simulink model "LIB_p2d_model_reference_R2021b"  (R2021b)
settings: Solver=FixedStepDiscrete  StartTime=0.0  StopTime=inf  FixedStep=dt  RelTol=1e-3
values from neighbouring files (symbols this model uses):
  Const = 0.065777522687874415    [LIB_p2d_dictionary.sldd]
  MatC = <binary blob, 30483 chars, not shown>    [LIB_p2d_dictionary.sldd]
  n1 = 5.0    [LIB_p2d_dictionary.sldd]    (also in P2D_run.m = mesh.n1)
  n2 = 2.0    [LIB_p2d_dictionary.sldd]    (also in P2D_run.m = mesh.n2)
  n3 = 5.0    [LIB_p2d_dictionary.sldd]    (also in P2D_run.m = mesh.n3)
  n4 = 5.0    [LIB_p2d_dictionary.sldd]
  ord = 2.0    [LIB_p2d_dictionary.sldd]    (also in P2D_run.m = mesh.ord)
undefined symbols (not defined in the file or in its folder): full
settings Model: DataDictionary=LIB_p2d_dictionary.sldd  EnableAccessToBaseWorkspace=off  Creator=simba  LastModifiedBy=simba
settings DebuggingCC: ParameterPrecisionLossMsg=none  UnconnectedInputMsg=none  UnconnectedOutputMsg=none  UnconnectedLineMsg=none
settings ModelReferenceCC: EnableRefExpFcnMdlSchedulingChecks=off
settings RTWCC: GPUComputeCapability=5.0  DLArmComputeVersion=20.02.1
settings ConfigComp: CovBoundaryAbsTol=1.0e-5

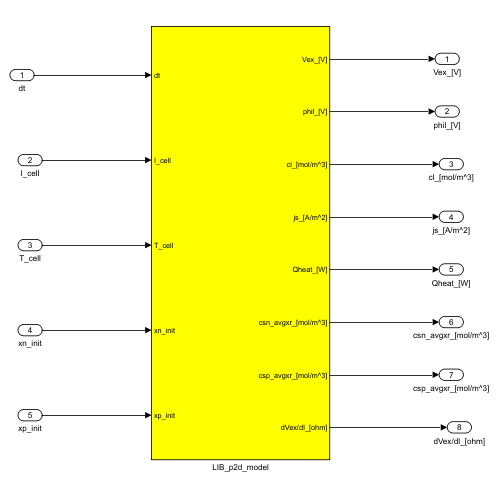
[thumbnail: Simulink's stored preview of the top-level diagram]
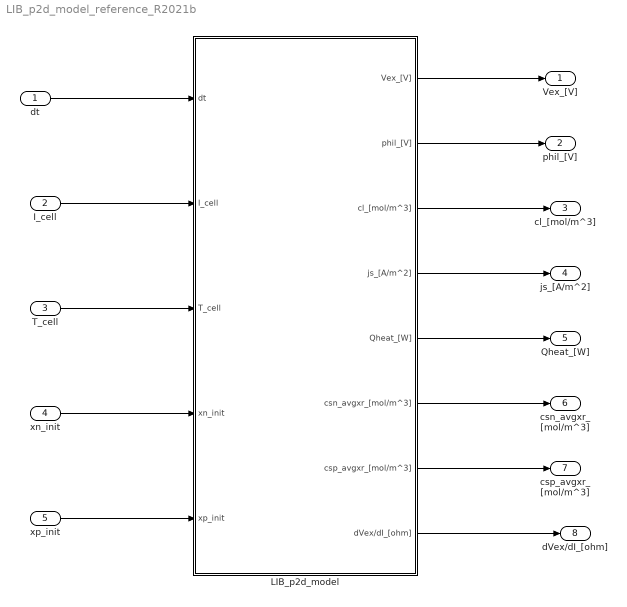
== system LIB_p2d_model_reference_R2021b ==
  dt : Inport  OutDataTypeStr=single
  I_cell : Inport  Port=2  OutDataTypeStr=single
  T_cell : Inport  Port=3  OutDataTypeStr=single
  xn_init : Inport  Port=4  OutDataTypeStr=single
  xp_init : Inport  Port=5  OutDataTypeStr=single
  LIB_p2d_model : Subsystem
  Vex_[V] : Outport
  phil_[V] : Outport  Port=2
  cl_[mol/m^3] : Outport  Port=3
  js_[A/m^2] : Outport  Port=4
  Qheat_[W] : Outport  Port=5
  csn_avgxr_[mol/m^3] : Outport  Port=6
  csp_avgxr_[mol/m^3] : Outport  Port=7
  dVex/dI_[ohm] : Outport  Port=8
  wires:
  dt/1 -> LIB_p2d_model/1(dt)
  I_cell/1 -> LIB_p2d_model/2(I_cell)
  T_cell/1 -> LIB_p2d_model/3(T_cell)
  xn_init/1 -> LIB_p2d_model/4(xn_init)
  xp_init/1 -> LIB_p2d_model/5(xp_init)
  LIB_p2d_model/1(Vex_[V]) -> Vex_[V]/1
  LIB_p2d_model/2(phil_[V]) -> phil_[V]/1
  LIB_p2d_model/3(cl_[mol/m^3]) -> cl_[mol/m^3]/1
  LIB_p2d_model/4(js_[A/m^2]) -> js_[A/m^2]/1
  LIB_p2d_model/5(Qheat_[W]) -> Qheat_[W]/1
  LIB_p2d_model/6(csn_avgxr_[mol/m^3]) -> csn_avgxr_[mol/m^3]/1
  LIB_p2d_model/7(csp_avgxr_[mol/m^3]) -> csp_avgxr_[mol/m^3]/1
  LIB_p2d_model/8(dVex/dI_[ohm]) -> dVex/dI_[ohm]/1

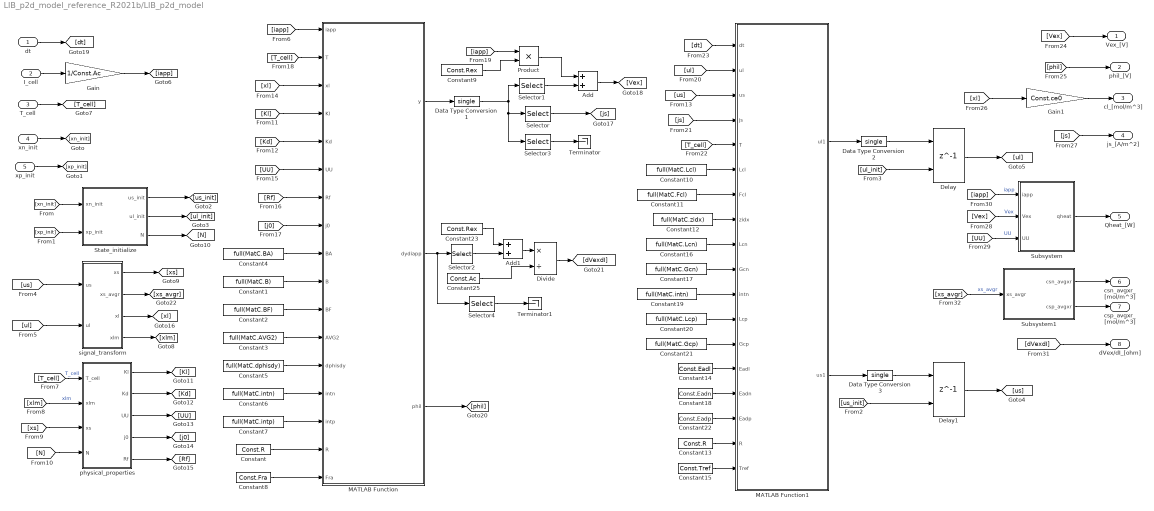
== system LIB_p2d_model_reference_R2021b/LIB_p2d_model ==
  dt : Inport
  I_cell : Inport  Port=2
  T_cell : Inport  Port=3
  xn_init : Inport  Port=4
  xp_init : Inport  Port=5
  Add : Sum
  Add1 : Sum
  Constant : Constant  Value=Const.R  OutDataTypeStr=single
  Constant1 : Constant  Value=full(MatC.B)  OutDataTypeStr=single
  Constant10 : Constant  Value=full(MatC.Lcl)  OutDataTypeStr=single
  Constant11 : Constant  Value=full(MatC.Fcl)  OutDataTypeStr=single
  Constant12 : Constant  Value=full(MatC.zidx)  OutDataTypeStr=uint8
  Constant13 : Constant  Value=Const.R  OutDataTypeStr=single
  Constant14 : Constant  Value=Const.Eadl  OutDataTypeStr=single
  Constant15 : Constant  Value=Const.Tref  OutDataTypeStr=single
  Constant16 : Constant  Value=full(MatC.Lcn)  OutDataTypeStr=single
  Constant17 : Constant  Value=full(MatC.Gcn)  OutDataTypeStr=single
  Constant18 : Constant  Value=Const.Eadn  OutDataTypeStr=single
  Constant19 : Constant  Value=full(MatC.intn)  VectorParams1D=off  OutDataTypeStr=single
  Constant2 : Constant  Value=full(MatC.BF)  OutDataTypeStr=single
  Constant20 : Constant  Value=full(MatC.Lcp)  OutDataTypeStr=single
  Constant21 : Constant  Value=full(MatC.Gcp)  OutDataTypeStr=single
  Constant22 : Constant  Value=Const.Eadp  OutDataTypeStr=single
  Constant23 : Constant  Value=Const.Rex  OutDataTypeStr=single
  Constant25 : Constant  Value=Const.Ac  OutDataTypeStr=single
  Constant3 : Constant  Value=full(MatC.AVG2)  OutDataTypeStr=single
  Constant4 : Constant  Value=full(MatC.BA)  OutDataTypeStr=single
  Constant5 : Constant  Value=full(MatC.dphisdy)  OutDataTypeStr=single
  Constant6 : Constant  Value=full(MatC.intn)  VectorParams1D=off  OutDataTypeStr=single
  Constant7 : Constant  Value=full(MatC.intp)  VectorParams1D=off  OutDataTypeStr=single
  Constant8 : Constant  Value=Const.Fra  OutDataTypeStr=single
  Constant9 : Constant  Value=Const.Rex  OutDataTypeStr=single
  Data Type Conversion1 : DataTypeConversion  OutDataTypeStr=single
  Data Type Conversion2 : DataTypeConversion  OutDataTypeStr=single
  Data Type Conversion3 : DataTypeConversion  OutDataTypeStr=single
  Delay : Delay  DelayLength=1  InitialConditionSource=Input port  InitialCondition=0
      settings: InputPortMap=u0,p4
  Delay1 : Delay  DelayLength=1  InitialConditionSource=Input port  InitialCondition=0
      settings: InputPortMap=u0,p4
  Divide : Product  Inputs=*/
  Gain : Gain  Gain=1/Const.Ac
  Gain1 : Gain  Gain=Const.ce0
  MATLAB Function : MATLAB Function  TreatAsAtomicUnit=on
  MATLAB Function1 : MATLAB Function  TreatAsAtomicUnit=on
  Product : Product
  Selector : Selector  IndexOptions=Index vector (dialog)  Indices=1:n1+n3  OutputSizes=1
  Selector1 : Selector  IndexOptions=Index vector (dialog)  Indices=n1+n3+2  OutputSizes=1
  Selector2 : Selector  IndexOptions=Index vector (dialog)  Indices=n1+n3+2  OutputSizes=1
  Selector3 : Selector  IndexOptions=Index vector (dialog)  Indices=n1+n3+3  OutputSizes=1
  Selector4 : Selector  IndexOptions=Index vector (dialog)  Indices=n1+n3+3  OutputSizes=1
  State_initialize : Subsystem
  Subsystem : Subsystem
  Subsystem1 : Subsystem
  Terminator : Terminator
  Terminator1 : Terminator
  physical_properties : Subsystem
  signal_transform : Subsystem
  Vex_[V] : Outport
  phil_[V] : Outport  Port=2
  cl_[mol/m^3] : Outport  Port=3
  js_[A/m^2] : Outport  Port=4
  Qheat_[W] : Outport  Port=5
  csn_avgxr_[mol/m^3] : Outport  Port=6
  csp_avgxr_[mol/m^3] : Outport  Port=7
  dVex/dI_[ohm] : Outport  Port=8
  wires:
  xn_init/1 -> [xn_init]
  xp_init/1 -> [xp_init]
  [xn_init] -> State_initialize/1(xn_init)
  [xp_init] -> State_initialize/2(xp_init)
  State_initialize/1(us_init) -> [us_init]
  State_initialize/2(ul_init) -> [ul_init]
  [us_init] -> Delay1/2
  [ul_init] -> Delay/2
  [us] -> signal_transform/1(us)
  [ul] -> signal_transform/2(ul)
  I_cell/1 -> Gain/1
  Gain/1 -> [iapp]
  T_cell/1 -> [T_cell]
  signal_transform/4(xlm) -> [xlm]
  [T_cell] -> physical_properties/1(T_cell)  "T_cell"
  [xlm] -> physical_properties/2(xlm)  "xlm"
  signal_transform/1(xs) -> [xs]
  [xs] -> physical_properties/3(xs)
  State_initialize/3(N) -> [N]
  [N] -> physical_properties/4(N)
  physical_properties/1(Kl) -> [Kl]
  physical_properties/2(Kd) -> [Kd]
  physical_properties/3(UU) -> [UU]
  physical_properties/4(j0) -> [j0]
  physical_properties/5(Rf) -> [Rf]
  [iapp] -> MATLAB Function/1(iapp)
  [Kl] -> MATLAB Function/4(Kl)
  Constant4/1 -> MATLAB Function/9(BA)
  Constant1/1 -> MATLAB Function/10(B)
  MATLAB Function/1(y) -> Data Type Conversion1/1
  Constant2/1 -> MATLAB Function/11(BF)
  [Kd] -> MATLAB Function/5(Kd)
  Constant3/1 -> MATLAB Function/12(AVG2)
  signal_transform/3(xl) -> [xl]
  [xl] -> MATLAB Function/3(xl)
  [UU] -> MATLAB Function/6(UU)
  Constant5/1 -> MATLAB Function/13(dphisdy)
  [Rf] -> MATLAB Function/7(Rf)
  Constant6/1 -> MATLAB Function/14(intn)
  Constant7/1 -> MATLAB Function/15(intp)
  [j0] -> MATLAB Function/8(j0)
  [T_cell] -> MATLAB Function/2(T)
  Constant/1 -> MATLAB Function/16(R)
  Constant8/1 -> MATLAB Function/17(Fra)
  Selector/1 -> [js]
  Constant9/1 -> Product/2
  [iapp] -> Product/1
  Product/1 -> Add/1
  Selector1/1 -> Add/2
  Add/1 -> [Vex]
  [ul] -> MATLAB Function1/2(ul)
  [us] -> MATLAB Function1/3(us)
  [js] -> MATLAB Function1/4(js)
  [T_cell] -> MATLAB Function1/5(T)
  Constant10/1 -> MATLAB Function1/6(Lcl)
  Constant11/1 -> MATLAB Function1/7(Fcl)
  Constant12/1 -> MATLAB Function1/8(zidx)
  Constant13/1 -> MATLAB Function1/17(R)
  Constant14/1 -> MATLAB Function1/14(Eadl)
  Constant15/1 -> MATLAB Function1/18(Tref)
  Constant16/1 -> MATLAB Function1/9(Lcn)
  Constant17/1 -> MATLAB Function1/10(Gcn)
  [dt] -> MATLAB Function1/1(dt)
  dt/1 -> [dt]
  Constant18/1 -> MATLAB Function1/15(Eadn)
  Constant19/1 -> MATLAB Function1/11(intn)
  Constant21/1 -> MATLAB Function1/13(Gcp)
  Constant20/1 -> MATLAB Function1/12(Lcp)
  Constant22/1 -> MATLAB Function1/16(Eadp)
  MATLAB Function1/1(ul1) -> Data Type Conversion2/1
  Delay/1 -> [ul]
  MATLAB Function1/2(us1) -> Data Type Conversion3/1
  Delay1/1 -> [us]
  Data Type Conversion1/1 -> Selector3/1, Selector/1, Selector1/1
  Data Type Conversion2/1 -> Delay/1
  Data Type Conversion3/1 -> Delay1/1
  [Vex] -> Vex_[V]/1
  MATLAB Function/3(phil) -> [phil]
  [phil] -> phil_[V]/1
  [xl] -> Gain1/1
  Gain1/1 -> cl_[mol/m^3]/1
  [js] -> js_[A/m^2]/1
  [iapp] -> Subsystem/1(iapp)  "iapp"
  [Vex] -> Subsystem/2(Vex)  "Vex"
  [UU] -> Subsystem/3(UU)  "UU"
  Subsystem/1(qheat) -> Qheat_[W]/1
  signal_transform/2(xs_avgr) -> [xs_avgr]
  [xs_avgr] -> Subsystem1/1(xs_avgr)  "xs_avgr"
  Subsystem1/1(csn_avgxr) -> csn_avgxr_[mol/m^3]/1
  Subsystem1/2(csp_avgxr) -> csp_avgxr_[mol/m^3]/1
  Selector2/1 -> Add1/2
  Constant23/1 -> Add1/1
  Add1/1 -> Divide/1
  Constant25/1 -> Divide/2
  Divide/1 -> [dVexdI]
  [dVexdI] -> dVex/dI_[ohm]/1
  Selector3/1 -> Terminator/1
  Selector4/1 -> Terminator1/1
  MATLAB Function/2(dydiapp) -> Selector4/1, Selector2/1

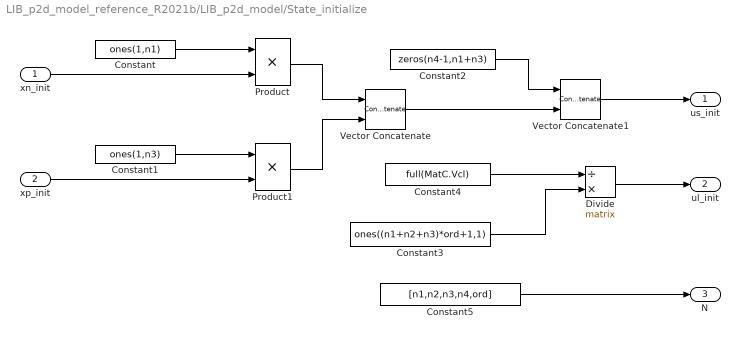
== system LIB_p2d_model_reference_R2021b/LIB_p2d_model/State_initialize ==
  xn_init : Inport
  xp_init : Inport  Port=2
  Constant : Constant  Value=ones(1,n1)  VectorParams1D=off  OutDataTypeStr=single
  Constant1 : Constant  Value=ones(1,n3)  VectorParams1D=off  OutDataTypeStr=single
  Constant2 : Constant  Value=zeros(n4-1,n1+n3)  VectorParams1D=off  OutDataTypeStr=single
  Constant3 : Constant  Value=ones((n1+n2+n3)*ord+1,1)  VectorParams1D=off  OutDataTypeStr=single
  Constant4 : Constant  Value=full(MatC.Vcl)  OutDataTypeStr=single
  Constant5 : Constant  Value=[n1,n2,n3,n4,ord]  OutDataTypeStr=uint8
  Divide : Product  Inputs=/*  Multiplication=Matrix(*)
  Product : Product
  Product1 : Product
  Vector Concatenate : Concatenate  Mode=Multidimensional array  ConcatenateDimension=2
  Vector Concatenate1 : Concatenate  Mode=Multidimensional array
  us_init : Outport
  ul_init : Outport  Port=2
  N : Outport  Port=3
  wires:
  Vector Concatenate1/1 -> us_init/1
  Constant/1 -> Product/1
  Constant1/1 -> Product1/1
  xp_init/1 -> Product1/2
  xn_init/1 -> Product/2
  Product1/1 -> Vector Concatenate/2
  Vector Concatenate/1 -> Vector Concatenate1/2
  Product/1 -> Vector Concatenate/1
  Constant2/1 -> Vector Concatenate1/1
  Constant3/1 -> Divide/2
  Constant4/1 -> Divide/1
  Divide/1 -> ul_init/1
  Constant5/1 -> N/1

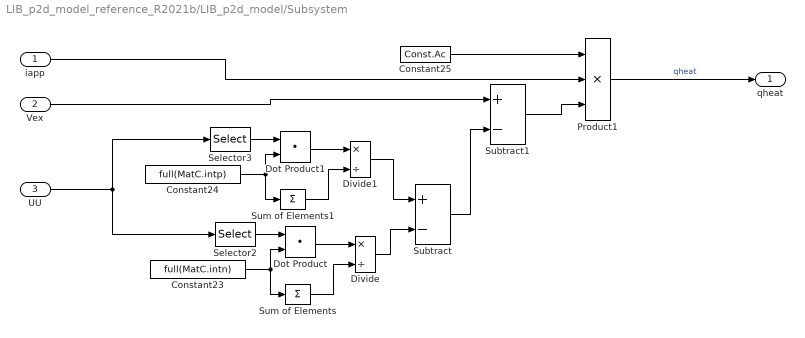
== system LIB_p2d_model_reference_R2021b/LIB_p2d_model/Subsystem ==
  iapp : Inport
  Vex : Inport  Port=2
  UU : Inport  Port=3
  Constant23 : Constant  Value=full(MatC.intn)  VectorParams1D=off  OutDataTypeStr=single
  Constant24 : Constant  Value=full(MatC.intp)  VectorParams1D=off  OutDataTypeStr=single
  Constant25 : Constant  Value=Const.Ac  OutDataTypeStr=single
  Divide : Product  Inputs=*/
  Divide1 : Product  Inputs=*/
  Dot Product : DotProduct  InputSameDT=on  OutDataTypeStr=Inherit: Inherit via internal rule
  Dot Product1 : DotProduct  InputSameDT=on  OutDataTypeStr=Inherit: Inherit via internal rule
  Product1 : Product  Inputs=3
  Selector2 : Selector  IndexOptions=Index vector (dialog)  Indices=1:n1  OutputSizes=1
  Selector3 : Selector  IndexOptions=Index vector (dialog)  Indices=n1+1:n1+n3  OutputSizes=1
  Subtract : Sum  Inputs=+-
  Subtract1 : Sum  Inputs=+-
  Sum of Elements : Sum  Inputs=+
  Sum of Elements1 : Sum  Inputs=+
  qheat : Outport
  wires:
  Constant25/1 -> Product1/1
  Subtract1/1 -> Product1/3
  Dot Product/1 -> Divide/1
  Product1/1 -> qheat/1  "qheat"
  Constant23/1 -> Dot Product/2, Sum of Elements/1
  Sum of Elements/1 -> Divide/2
  Selector2/1 -> Dot Product/1
  UU/1 -> Selector3/1, Selector2/1
  Sum of Elements1/1 -> Divide1/2
  Vex/1 -> Subtract1/1
  Subtract/1 -> Subtract1/2
  Selector3/1 -> Dot Product1/1
  Constant24/1 -> Dot Product1/2, Sum of Elements1/1
  Dot Product1/1 -> Divide1/1
  Divide1/1 -> Subtract/1
  Divide/1 -> Subtract/2
  iapp/1 -> Product1/2

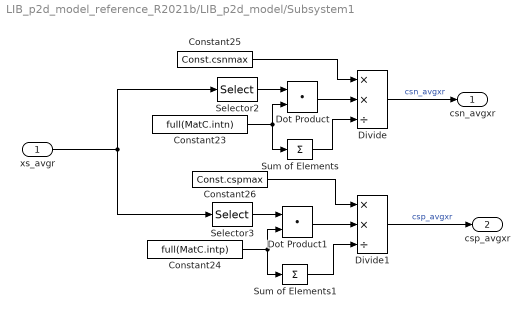
== system LIB_p2d_model_reference_R2021b/LIB_p2d_model/Subsystem1 ==
  xs_avgr : Inport
  Constant23 : Constant  Value=full(MatC.intn)  VectorParams1D=off  OutDataTypeStr=single
  Constant24 : Constant  Value=full(MatC.intp)  VectorParams1D=off  OutDataTypeStr=single
  Constant25 : Constant  Value=Const.csnmax  OutDataTypeStr=single
  Constant26 : Constant  Value=Const.cspmax  OutDataTypeStr=single
  Divide : Product  Inputs=**/
  Divide1 : Product  Inputs=**/
  Dot Product : DotProduct  InputSameDT=on  OutDataTypeStr=Inherit: Inherit via internal rule
  Dot Product1 : DotProduct  InputSameDT=on  OutDataTypeStr=Inherit: Inherit via internal rule
  Selector2 : Selector  IndexOptions=Index vector (dialog)  Indices=1:n1  OutputSizes=1
  Selector3 : Selector  IndexOptions=Index vector (dialog)  Indices=n1+1:n1+n3  OutputSizes=1
  Sum of Elements : Sum  Inputs=+
  Sum of Elements1 : Sum  Inputs=+
  csn_avgxr : Outport
  csp_avgxr : Outport  Port=2
  wires:
  Constant26/1 -> Divide1/1
  Constant24/1 -> Dot Product1/2, Sum of Elements1/1
  Dot Product/1 -> Divide/2
  Sum of Elements1/1 -> Divide1/3
  Constant23/1 -> Dot Product/2, Sum of Elements/1
  Sum of Elements/1 -> Divide/3
  Selector2/1 -> Dot Product/1
  Selector3/1 -> Dot Product1/1
  xs_avgr/1 -> Selector3/1, Selector2/1
  Dot Product1/1 -> Divide1/2
  Constant25/1 -> Divide/1
  Divide1/1 -> csp_avgxr/1  "csp_avgxr"
  Divide/1 -> csn_avgxr/1  "csn_avgxr"

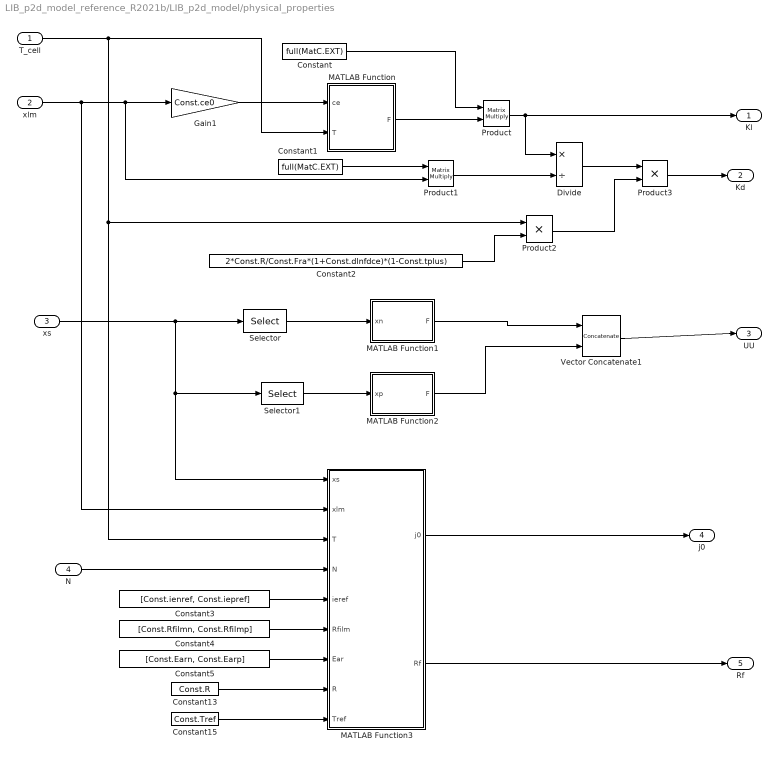
== system LIB_p2d_model_reference_R2021b/LIB_p2d_model/physical_properties ==
  T_cell : Inport
  xlm : Inport  Port=2
  xs : Inport  Port=3
  N : Inport  Port=4
  Constant : Constant  Value=full(MatC.EXT)  OutDataTypeStr=single
  Constant1 : Constant  Value=full(MatC.EXT)  OutDataTypeStr=single
  Constant13 : Constant  Value=Const.R  OutDataTypeStr=single
  Constant15 : Constant  Value=Const.Tref  OutDataTypeStr=single
  Constant2 : Constant  Value=2*Const.R/Const.Fra*(1+Const.dlnfdce)*(1-Const.tplus)  OutDataTypeStr=single
  Constant3 : Constant  Value=[Const.ienref, Const.iepref]  OutDataTypeStr=single
  Constant4 : Constant  Value=[Const.Rfilmn, Const.Rfilmp]  OutDataTypeStr=single
  Constant5 : Constant  Value=[Const.Earn, Const.Earp]  OutDataTypeStr=single
  Divide : Product  Inputs=*/
  Gain1 : Gain  Gain=Const.ce0
  MATLAB Function : MATLAB Function  TreatAsAtomicUnit=on
  MATLAB Function1 : MATLAB Function  TreatAsAtomicUnit=on
  MATLAB Function2 : MATLAB Function  TreatAsAtomicUnit=on
  MATLAB Function3 : MATLAB Function  TreatAsAtomicUnit=on
  Product : Product  Multiplication=Matrix(*)
  Product1 : Product  Multiplication=Matrix(*)
  Product2 : Product
  Product3 : Product
  Selector : Selector  IndexOptions=Index vector (dialog)  Indices=1:n1  OutputSizes=1
  Selector1 : Selector  IndexOptions=Index vector (dialog)  Indices=n1+1:n1+n3  OutputSizes=1
  Vector Concatenate1 : Concatenate  Mode=Multidimensional array
  Kl : Outport
  Kd : Outport  Port=2
  UU : Outport  Port=3
  j0 : Outport  Port=4
  Rf : Outport  Port=5
  wires:
  Gain1/1 -> MATLAB Function/1(ce)
  T_cell/1 -> MATLAB Function3/3(T), Product2/1, MATLAB Function/2(T)
  MATLAB Function/1(F) -> Product/2
  xlm/1 -> MATLAB Function3/2(xlm), Product1/2, Gain1/1
  Constant/1 -> Product/1
  Constant1/1 -> Product1/1
  Product1/1 -> Divide/2
  Product/1 -> Divide/1, Kl/1
  Constant2/1 -> Product2/2
  Divide/1 -> Product3/1
  Product2/1 -> Product3/2
  Product3/1 -> Kd/1
  xs/1 -> Selector1/1, MATLAB Function3/1(xs), Selector/1
  Selector/1 -> MATLAB Function1/1(xn)
  MATLAB Function1/1(F) -> Vector Concatenate1/1
  Selector1/1 -> MATLAB Function2/1(xp)
  MATLAB Function2/1(F) -> Vector Concatenate1/2
  Vector Concatenate1/1 -> UU/1
  N/1 -> MATLAB Function3/4(N)
  Constant3/1 -> MATLAB Function3/5(ieref)
  Constant4/1 -> MATLAB Function3/6(Rfilm)
  MATLAB Function3/1(j0) -> j0/1
  MATLAB Function3/2(Rf) -> Rf/1
  Constant5/1 -> MATLAB Function3/7(Ear)
  Constant13/1 -> MATLAB Function3/8(R)
  Constant15/1 -> MATLAB Function3/9(Tref)

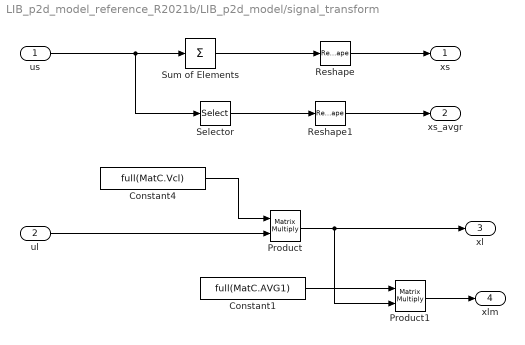
== system LIB_p2d_model_reference_R2021b/LIB_p2d_model/signal_transform ==
  us : Inport
  ul : Inport  Port=2
  Constant1 : Constant  Value=full(MatC.AVG1)  OutDataTypeStr=single
  Constant4 : Constant  Value=full(MatC.Vcl)  OutDataTypeStr=single
  Product : Product  Multiplication=Matrix(*)
  Product1 : Product  Multiplication=Matrix(*)
  Reshape : Reshape  OutputDimensionality=Column vector (2-D)
  Reshape1 : Reshape  OutputDimensionality=Column vector (2-D)
  Selector : Selector  NumberOfDimensions=2  InputPortWidth=3  IndexOptions=Index vector (dialog),Select all  Indices=n4,1  OutputSizes=1,1
  Sum of Elements : Sum  Inputs=+  CollapseMode=Specified dimension
  xs : Outport
  xs_avgr : Outport  Port=2
  xl : Outport  Port=3
  xlm : Outport  Port=4
  wires:
  us/1 -> Selector/1, Sum of Elements/1
  Sum of Elements/1 -> Reshape/1
  Reshape/1 -> xs/1
  Constant4/1 -> Product/1
  ul/1 -> Product/2
  Product/1 -> Product1/2, xl/1
  Constant1/1 -> Product1/1
  Product1/1 -> xlm/1
  Selector/1 -> Reshape1/1
  Reshape1/1 -> xs_avgr/1

== matlab function LIB_p2d_model_reference_R2021b/LIB_p2d_model/physical_properties/MATLAB Function1 ==
  data: xn input; F output
function F=Un(xn)%Open circuit potential of negative electrode [V]
b=[0.164,0.48,90,0.01,0.025,300,0.136,0.032,100,0.161,0.032,50,0.22,0.032,80,0.505,0.1,90,0.965];
Un_const=b(1);
Un_exp1=b(2)*exp(-b(3)*(xn-b(4)));
Un_atan1=-b(5)/pi*atan(b(6)*(xn-b(7)));
Un_atan2=-b(8)/pi*atan(b(9)*(xn-b(10)));
Un_atan3=-b(11)/pi*atan(b(12)*(xn-b(13)));
Un_atan4=-b(14)/pi*atan(b(15)*(xn-b(16)));
Un_exp2=-b(17)*exp(b(18)*(xn-b(19)));
F=Un_const+Un_exp1+Un_atan1+Un_atan2+Un_atan3+Un_atan4+Un_exp2;
end

== matlab function LIB_p2d_model_reference_R2021b/LIB_p2d_model/physical_properties/MATLAB Function ==
  data: ce input; F output; T input
function F=kappa(ce,T)%Electrolyte conductivity (S/m)
F=(3.45*exp(-798/T)*(ce/1000).^3-48.5*exp(-1080/T)*(ce/1000).^2+244*exp(-1440/T)*(ce/1000));
end

== matlab function LIB_p2d_model_reference_R2021b/LIB_p2d_model/physical_properties/MATLAB Function2 ==
  data: xp input; F output
function F=Up(xp)%Open circuit potential of positive electrode [V]
b=[3.67287671914126,0.0392134821245406,0.999470977852800,0.419937084206002,12.8799319870686,-47.2135901049774,64.6252944547241,-40.4701303771546,10.1693381074356;];
b_Nernst=b(1:3);
OCP_charge_Nernst=b_Nernst(1)+b_Nernst(2)*log(b_Nernst(3)-xp);
b_poly=b(4:end);
order=length(b_poly);
dOCP_charge_fit=0*xp;
for i=1:order
    dOCP_charge_fit=dOCP_charge_fit+b_poly(order+1-i)*xp.^(i);
end
F=OCP_charge_Nernst+dOCP_charge_fit;
end

== matlab function LIB_p2d_model_reference_R2021b/LIB_p2d_model/physical_properties/MATLAB Function3 ==
  data: xs input; j0 output; xlm input; T input; N input; ieref input; Rf output; Rfilm input; Ear input; R input; Tref input
function [j0, Rf] = j0_Rf(xs, xlm, T, N, ieref, Rfilm, Ear, R, Tref)
n1 = uint8(N(1));
n2 = uint8(N(2));
n3 = uint8(N(3));
j0 = xs*0;
j0(1:n1) = ieref(1)*sqrt(xs(1:n1).*(1-xs(1:n1)).*xlm(1:n1))*exp(-Ear(1)/R*(1/T-1/Tref));
j0(n1+1:n1+n3) = ieref(2)*sqrt(xs(n1+1:n1+n3).*(1-xs(n1+1:n1+n3)).*xlm(n1+n2+1:n1+n2+n3))*exp(-Ear(2)/R*(1/T-1/Tref));
Rf = xs*0;
Rf(1:n1) = ones(n1,1)*Rfilm(1);
Rf(n1+1:n1+n3) = ones(n3,1)*Rfilm(2);
end

== matlab function LIB_p2d_model_reference_R2021b/LIB_p2d_model/MATLAB Function ==
  data: iapp input; T input; xl input; y output; Kl input; Kd input; UU input; Rf input; j0 input; BA input; B input; BF input; AVG2 input; dphisdy input; intn input; intp input; R input; Fra input; dydiapp output; phil output
function [y, dydiapp, phil] = charge_conservation(iapp, T, xl, Kl, Kd, UU, Rf, j0, BA, B, BF, AVG2, dphisdy, intn, intp, R, Fra)
n1 = uint8(length(intn));
n13 = uint8(size(BF,2));
%% Charge conservation equations
MM1 = BA*(Kl.*B);
MM1(1,:) = 0;
MM1(1,1) = 1;
BF(1,:) = 0;
MM2 = BA*(Kd.*B);
MM2(1,:) = 0;
KK = MM1\BF;
ff = (MM1\MM2)*xl;
dphildy = single(zeros(n13, n13+3));
dphildy(:,1:n13) = AVG2*(KK);
dphildy(:,1+n13) = 1;
feta = - AVG2*ff - UU;
dphisldy = single(zeros(n13, n13+3));
dphisldy(:,1:n13+2) = dphisdy - dphildy(:,1:n13+2);
detady = dphisldy;
detady(:,1:n13) = detady(:,1:n13) - diag(Rf);

%% Inilization
eta_avg = single([0,0]);
eta_avg(1) = asinh(-iapp/(2*intn*j0(1:n1)));
eta_avg(2) = asinh(iapp/(2*intp*j0(n1+1:n13)));
Hyb_corr = single([1,1]);

if abs(eta_avg(1))>1e-4
    Hyb_corr(1) = sinh(eta_avg(1))/eta_avg(1);
end

if abs(eta_avg(2))>1e-4
    Hyb_corr(2) = sinh(eta_avg(2))/eta_avg(2);
end

j0_Hyb = j0;
j0_Hyb(1:n1) = j0_Hyb(1:n1)*Hyb_corr(1);
j0_Hyb(n1+1:n13) = j0_Hyb(n1+1:n13)*Hyb_corr(2);

Jac = single(zeros(n13+3,n13+3));
Jac(1:n13,1:n13) = diag(Rf + R*T./(j0_Hyb*Fra));
Jac(1:n13,:) = Jac(1:n13,:) - dphisldy;
Jac(n13+1,1:n1) = intn;
Jac(n13+1,n1+1:n13) = intp;
Jac(n13+2,1:n1) = intn;
Jac(n13+2,n1+1:n13) = -intp;
Jac(n13+2,n13+3) = 2;
Jac(n13+3,n13+3) = 1;

Res = single(zeros(n13+3,1));
Res(1:n13) = feta;
Res(n13+3) = iapp;
y = Jac\Res;

dydiapp  = Jac(:,:)\[zeros(n13+2,1);1];

%%
eta = detady*y + feta;
jexpf = j0.*exp(0.5*Fra/R/T*eta);
jexpr = j0.*exp(-0.5*Fra/R/T*eta);
deta = single([0,0]);

A = intn*jexpf(1:n1);
B = intn*jexpr(1:n1);
X = (-iapp + sqrt(iapp^2 + 4*A*B))/(2*A);
y(1:n1) = jexpf(1:n1)*X - jexpr(1:n1)/X;
deta(1) = log(X)*(R*T/(0.5*Fra));

A = intp*jexpf(n1+1:n13);
B = intp*jexpr(n1+1:n13);
X = (iapp + sqrt(iapp^2 + 4*A*B))/(2*A);
y(n1+1:n13) = jexpf(n1+1:n13)*X - jexpr(n1+1:n13)/X;
deta(2) = log(X)*(R*T/(0.5*Fra));

y(n13+1) = y(n13+1) - deta(1);
y(n13+2) = y(n13+2) + deta(2) - deta(1);

%% Evaluate electrolyte potential
phil = KK*y(1:n13) + ff + y(n13+1);
end

== matlab function LIB_p2d_model_reference_R2021b/LIB_p2d_model/MATLAB Function1 ==
  data: dt input; ul1 output; ul input; us input; js input; T input; Lcl input; Fcl input; zidx input; Lcn input; Gcn input; intn input; Lcp input; Gcp input; Eadl input; Eadn input; Eadp input; R input; Tref input; us1 output
function [ul1, us1] = mass_transfer(dt, ul, us, js, T, Lcl, Fcl, zidx, Lcn, Gcn, intn, Lcp, Gcp, Eadl, Eadn, Eadp, R, Tref)
%% Basic settings
n1 = uint8(length(intn));
n4 = uint8(length(Lcn));
n13 = uint8(size(js,1));

ul1 = ul;
us1 = us;
%% Electrolyte diffusion
fcl = Fcl*js;
nn = uint8(size(Fcl,1));
for ii = 1:nn
    lambda = Lcl(ii)*exp(-Eadl/R*(1/T-1/Tref));
    if ii ~= zidx
        ul1(ii) = ul(ii)*exp(-lambda*dt) + (1 - exp(-lambda*dt))/lambda*fcl(ii);
    else
        ul1(ii) = ul(ii) + fcl(ii)*dt;
    end
end

%% Anode particle diffusion
lambda = Lcn*exp(-Eadn/R*(1/T-1/Tref));
for jj = 1:n1    
    for ii = 1:n4-1
        us1(ii,jj) = us(ii,jj)*exp(-lambda(ii)*dt) + (1 - exp(-lambda(ii)*dt))/lambda(ii)*Gcn(ii)*js(jj);
    end 
    us1(n4,jj) = us(n4,jj) + dt*Gcn(n4)*js(jj);
end

%% Cathode particle diffusion
lambda = Lcp*exp(-Eadp/R*(1/T-1/Tref));
for jj = n1+1:n13    
    for ii = 1:n4-1
        us1(ii,jj) = us(ii,jj)*exp(-lambda(ii)*dt) + (1 - exp(-lambda(ii)*dt))/lambda(ii)*Gcp(ii)*js(jj);
    end 
    us1(n4,jj) = us(n4,jj) + dt*Gcp(ii+1)*js(jj);
end

end
